simulink model "quad_sim_pyramid_formation"  (R2017b)
settings: Solver=VariableStepAuto  StartTime=0.0  StopTime=300  FixedStep=0.025  MaxStep=0.03  MinStep=0.02  RelTol=1e-3  EnableMultiTasking=on
InitFcn:
  | time_to_enable=250
  | 
  | setup_gains
  | % --- Outer loop gains --------
  | %P_X=9.44;   I_X=0.23;  D_X=2.36;
  | %P_Y=9.33;   I_Y=0.18;  D_Y=1.54;
  | % --------------------------
  | 
  | %CARLA TUNNED PID
  | %P_Z = 51.037;       I_Z = 43.051;        D_Z = 11.771;
  | %P_Z = 0.5;       I_Z = 0.15;        D_Z = 0.2;
  | %P_Z = 32.55;       I_Z = 9.82;        D_Z = 4.65 ;
  | 
  | global clientID;
  | clientID=-1;
values from neighbouring files (symbols this model uses):
  End_POS_pyramid = End_POS_pyramid*0.9995    [sim_formation_syscon.m]    (also in sim_formation_syscon_vel.m = End_POS_pyramid*0.999; structure_assembly.m = End_POS_pyramid*0.995)
undefined symbols (not defined in the file or in its folder): Kd_az, Kd_px, Kd_py, Kd_pz, Kd_vx, Kd_vy, Kd_vz, Ki_az, Ki_px, Ki_py, Ki_pz, Ki_vx, Ki_vy, Ki_vz, Kp_az, Kp_px, Kp_py, Kp_pz, Kp_vx, Kp_vy, Kp_vz, Start_POS, W, X, Y, Z
libraries: robotlib x27, dspsigops x27, simulink x27, dspindex x9
(part 3 of 3)

== system quad_sim_pyramid_formation/Quadrotor 5/Quadrirrotor Communication ==
  roll : Inport
  pitch : Inport  Port=2
  yaw : Inport  Port=3
  throttle : Inport  Port=4
  Blank Message : robotlib/Blank Message  SourceLibraryInfo=This block requires Robotics System Toolbox  messageType=geometry_msgs/Quaternion  SampleTime=inf
      settings: SourceProductBaseCode=RO
  Bus Assignment1 : BusAssignment  DialogController=Simulink.DDGSource_BusAssignment  AssignedSignals=X,Y,Z,W
  Bus Selector1 : BusSelector  OutputSignals=Data
  Data Type Conversion : DataTypeConversion  OutDataTypeStr=double
  Multiport Selector : dspindex/Multiport Selector  rowsOrCols=Rows  idxCellArray={ 1,2,3,4,5,6,7,8,9}  idxErrMode=Generate Error
  Publish2 : robotlib/Publish  SourceLibraryInfo=This block requires Robotics System Toolbox  topicSource=Specify your own  topic=/commands_attitude_5  messageType=geometry_msgs/Quaternion  messageQueueLength=105
      settings: SourceProductBaseCode=RO
  Subscribe : robotlib/Subscribe  SourceLibraryInfo=This block requires Robotics System Toolbox  topicSource=Specify your own  topic=/quadrotor_states_5  messageType=std_msgs/Float32MultiArray  sampleTime=-1  messageQueueLength=51
      settings: SourceProductBaseCode=RO
  Terminator : Terminator
  quad_pos_x : Outport
  quad_pos_y : Outport  Port=2
  quad_pos_z : Outport  Port=3
  quad_vel_x : Outport  Port=4
  quad_vel_y : Outport  Port=5
  quad_vel_z : Outport  Port=6
  quad_acc_x : Outport  Port=7
  quad_acc_y : Outport  Port=8
  quad_acc_z : Outport  Port=9
  wires:
  Blank Message/1 -> Bus Assignment1/1
  Subscribe/1 -> Terminator/1
  Subscribe/2 -> Bus Selector1/1
  Bus Assignment1/1 -> Publish2/1
  Multiport Selector/1 -> quad_pos_x/1
  Multiport Selector/2 -> quad_pos_y/1
  Multiport Selector/3 -> quad_pos_z/1
  Multiport Selector/4 -> quad_vel_x/1
  Multiport Selector/5 -> quad_vel_y/1
  Multiport Selector/6 -> quad_vel_z/1
  Multiport Selector/7 -> quad_acc_x/1
  Multiport Selector/8 -> quad_acc_y/1
  Multiport Selector/9 -> quad_acc_z/1
  Data Type Conversion/1 -> Multiport Selector/1
  Bus Selector1/1 -> Data Type Conversion/1  "<Data>"
  throttle/1 -> Bus Assignment1/5
  yaw/1 -> Bus Assignment1/4
  pitch/1 -> Bus Assignment1/3
  roll/1 -> Bus Assignment1/2

== system quad_sim_pyramid_formation/Quadrotor 5/Subsystem1 ==
  desired : Inport
  actual : Inport  Port=2
  roll_in : Inport  Port=3
  pitch_in : Inport  Port=4
  yaw_in : Inport  Port=5
  height_in : Inport  Port=6
  Clock : Clock
  Compare To Constant : simulink/Logic and Bit Operations/Compare To Constant  relop=<  const=0.5  OutDataTypeStr=boolean
  Compare To Constant1 : simulink/Logic and Bit Operations/Compare To Constant  relop=<=  const=0.025  OutDataTypeStr=boolean
  Compare To Zero : simulink/Logic and Bit Operations/Compare To Zero  relop=<=  OutDataTypeStr=boolean
  Constant : Constant  Value=0
  Constant1 : Constant
  Data Store Memory : DataStoreMemory  DataStoreName=waypoints_reached5  ShowAdditionalParam=off  OutDataTypeStr=boolean
  Data Store Read{,1..4} (5 alike) : DataStoreRead  DataStoreName=waypoints_reached5
  Data Store Write : DataStoreWrite  DataStoreName=waypoints_reached5
  Demux : Demux  Outputs=3
  Fcn : Fcn  Expr=sqrt(u(1)^2+u(2)^2+u(3)^2)
  Logical Operator : Logic  AllPortsSameDT=off  OutDataTypeStr=boolean
  Mux8 : Mux  Inputs=3
  Sum1 : Sum  Inputs=+-
  Switch{,1..4} (5 alike) : Switch  Criteria=u2 > Threshold  Threshold=0.5
  Switch5 : Switch  Criteria=u2 > Threshold  Threshold=time_to_enable
  "angle " : Constant  Value=0
  angle 1 : Constant  Value=0
  angle 2 : Constant  Value=0
  angle 3 : Constant  Value=-1
  roll_out : Outport
  pitch_out : Outport  Port=2
  yaw_out : Outport  Port=3
  height_out : Outport  Port=4
  wires:
  roll_in/1 -> Switch1/3
  pitch_in/1 -> Switch2/3
  angle 2/1 -> Switch3/1
  yaw_in/1 -> Switch3/3
  "angle "/1 -> Switch1/1
  angle 1/1 -> Switch2/1
  height_in/1 -> Switch4/3
  Switch2/1 -> pitch_out/1
  Switch1/1 -> roll_out/1
  Demux/2 -> Mux8/2
  Demux/3 -> Switch5/1, Mux8/3
  Logical Operator/1 -> Switch/3
  Compare To Constant/1 -> Logical Operator/1
  Compare To Constant1/1 -> Logical Operator/2
  Sum1/1 -> Fcn/1
  Fcn/1 -> Compare To Constant1/1
  Mux8/1 -> Sum1/1
  Compare To Zero/1 -> Switch/1
  Data Store Read2/1 -> Switch2/2
  Data Store Read4/1 -> Switch4/2
  Data Store Read1/1 -> Switch1/2
  Switch/1 -> Data Store Write/1
  Data Store Read3/1 -> Switch3/2
  angle 3/1 -> Switch4/1
  Switch3/1 -> yaw_out/1
  Switch4/1 -> height_out/1
  Data Store Read/1 -> Switch/2
  Constant/1 -> Compare To Zero/1
  Demux/1 -> Mux8/1
  desired/1 -> Demux/1
  actual/1 -> Sum1/2
  Clock/1 -> Switch5/2
  Constant1/1 -> Switch5/3
  Switch5/1 -> Compare To Constant/1

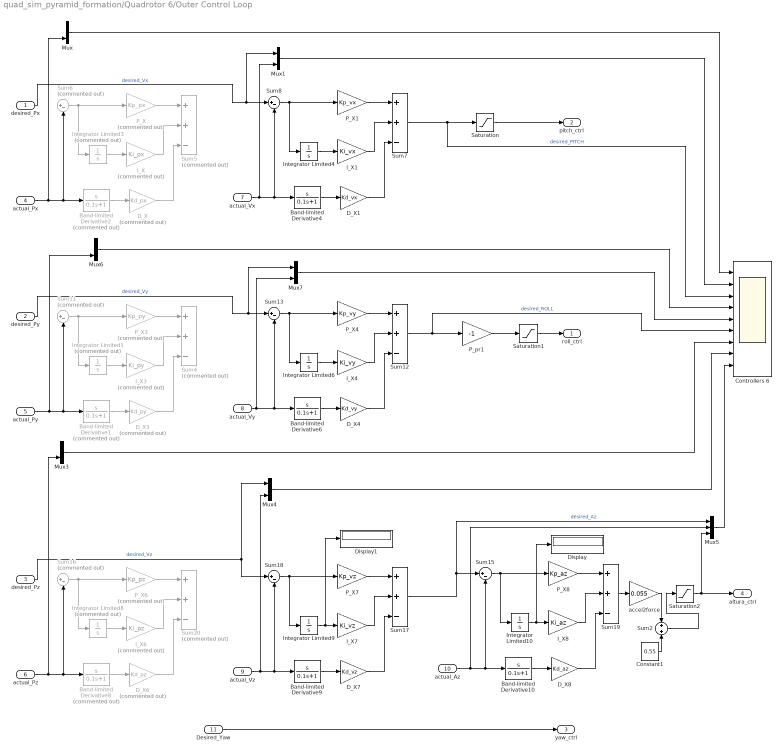
== system quad_sim_pyramid_formation/Quadrotor 6/Outer Control Loop ==
  desired_Px : Inport
  desired_Py : Inport  Port=2
  desired_Pz : Inport  Port=3
  actual_Px : Inport  Port=4
  actual_Py : Inport  Port=5
  actual_Pz : Inport  Port=6
  actual_Vx : Inport  Port=7
  actual_Vy : Inport  Port=8
  actual_Vz : Inport  Port=9
  actual_Az : Inport  Port=10
  Desired_Yaw : Inport  Port=11
  Band-limited Derivative1 : TransferFcn  Commented=on  Numerator=[1 0]  Denominator=[0.1 1]
  Band-limited Derivative{4,6,9..10} (4 alike) : TransferFcn  Numerator=[1 0]  Denominator=[0.1 1]
  Band-limited Derivative2 : TransferFcn  Commented=on  Numerator=[1 0]  Denominator=[0.1 1]
  Band-limited Derivative8 : TransferFcn  Commented=on  Numerator=[1 0]  Denominator=[0.1 1]
  Constant1 : Constant  Value=0.55
  Controllers 6 : Scope  NumInputPorts=9
  D_X : Gain  Commented=on  Gain=Kd_px
  D_X1 : Gain  Gain=Kd_vx
  D_X3 : Gain  Commented=on  Gain=Kd_py
  D_X4 : Gain  Gain=Kd_vy
  D_X6 : Gain  Commented=on  Gain=Kd_pz
  D_X7 : Gain  Gain=Kd_vz
  D_X8 : Gain  Gain=Kd_az
  Display : Display
  Display1 : Display
  I_X : Gain  Commented=on  Gain=Ki_px
  I_X1 : Gain  Gain=Ki_vx
  I_X3 : Gain  Commented=on  Gain=Ki_py
  I_X4 : Gain  Gain=Ki_vy
  I_X6 : Gain  Commented=on  Gain=Ki_pz
  I_X7 : Gain  Gain=Ki_vz
  I_X8 : Gain  Gain=Ki_az
  Integrator Limited1 : Integrator  Commented=on  LimitOutput=on  UpperSaturationLimit=100  LowerSaturationLimit=-100
  Integrator Limited10 : Integrator  LimitOutput=on  UpperSaturationLimit=1000  LowerSaturationLimit=-1000
  Integrator Limited3 : Integrator  Commented=on  LimitOutput=on  UpperSaturationLimit=100  LowerSaturationLimit=-100
  Integrator Limited4 : Integrator  LimitOutput=on  UpperSaturationLimit=100  LowerSaturationLimit=-100
  Integrator Limited6 : Integrator  LimitOutput=on  UpperSaturationLimit=100  LowerSaturationLimit=-100
  Integrator Limited8 : Integrator  Commented=on  LimitOutput=on  UpperSaturationLimit=1000  LowerSaturationLimit=-1000
  Integrator Limited9 : Integrator  LimitOutput=on  UpperSaturationLimit=1000  LowerSaturationLimit=-1000
  Mux{,1,3..4,6..7} (6 alike) : Mux  Inputs=2
  Mux5 : Mux  Inputs=3
  P_X : Gain  Commented=on  Gain=Kp_px
  P_X1 : Gain  Gain=Kp_vx
  P_X3 : Gain  Commented=on  Gain=Kp_py
  P_X4 : Gain  Gain=Kp_vy
  P_X6 : Gain  Commented=on  Gain=Kp_pz
  P_X7 : Gain  Gain=Kp_vz
  P_X8 : Gain  Gain=Kp_az
  P_pr1 : Gain  Gain=-1
  Saturation : Saturate  UpperLimit=5  LowerLimit=-5
  Saturation1 : Saturate  UpperLimit=5  LowerLimit=-5
  Saturation2 : Saturate  UpperLimit=10  LowerLimit=0
  Sum11 : Sum  Commented=on  Inputs=|+-
  Sum{7,12,17,19} (4 alike) : Sum  Inputs=++-
  Sum{8,13,15,18} (4 alike) : Sum  Inputs=|+-
  Sum16 : Sum  Commented=on  Inputs=|+-
  Sum2 : Sum  Inputs=+|+
  Sum20 : Sum  Commented=on  Inputs=++-
  Sum4 : Sum  Commented=on  Inputs=++-
  Sum5 : Sum  Commented=on  Inputs=++-
  Sum6 : Sum  Commented=on  Inputs=|+-
  accel2force : Gain  Gain=0.055
  roll_ctrl : Outport
  pitch_ctrl : Outport  Port=2
  yaw_ctrl : Outport  Port=3
  altura_ctrl : Outport  Port=4
  wires:
  Saturation1/1 -> roll_ctrl/1
  Saturation/1 -> pitch_ctrl/1
  P_pr1/1 -> Saturation1/1
  Mux7/1 -> Controllers 6/5
  Mux6/1 -> Controllers 6/4
  actual_Vy/1 -> Mux7/2, Sum13/2, Band-limited Derivative6/1
  actual_Py/1 -> Mux6/2, Band-limited Derivative1/1, Sum11/2
  Constant1/1 -> Sum2/2
  accel2force/1 -> Sum2/1
  Sum2/1 -> Saturation2/1
  Sum19/1 -> accel2force/1
  Mux5/1 -> Controllers 6/9
  Mux4/1 -> Controllers 6/8
  Mux3/1 -> Controllers 6/7
  Sum17/1 -> Sum15/1, Mux5/1  "desired_Az"
  actual_Az/1 -> Sum15/2, Band-limited Derivative10/1, Mux5/2
  desired_Pz/1 -> Sum18/1, Mux4/1  "desired_Vz"
  actual_Vz/1 -> Band-limited Derivative9/1, Sum18/2, Mux4/2
  Mux1/1 -> Controllers 6/2
  Mux/1 -> Controllers 6/1
  I_X8/1 -> Sum19/2
  Band-limited Derivative10/1 -> D_X8/1
  D_X8/1 -> Sum19/3
  P_X8/1 -> Sum19/1
  Integrator Limited10/1 -> I_X8/1, Display/1
  Sum15/1 -> P_X8/1, Integrator Limited10/1
  I_X7/1 -> Sum17/2
  Band-limited Derivative9/1 -> D_X7/1
  D_X7/1 -> Sum17/3
  P_X7/1 -> Sum17/1
  Integrator Limited9/1 -> I_X7/1, Display1/1
  Sum18/1 -> Integrator Limited9/1, P_X7/1
  I_X6/1 -> Sum20/2
  Band-limited Derivative8/1 -> D_X6/1
  actual_Pz/1 -> Sum16/2, Band-limited Derivative8/1, Mux3/2
  D_X6/1 -> Sum20/3
  P_X6/1 -> Sum20/1
  Integrator Limited8/1 -> I_X6/1
  Sum16/1 -> P_X6/1, Integrator Limited8/1
  Sum12/1 -> Controllers 6/6, P_pr1/1  "desired_ROLL"
  desired_Py/1 -> Mux7/1, Sum13/1  "desired_Vy"
  I_X4/1 -> Sum12/2
  Band-limited Derivative6/1 -> D_X4/1
  D_X4/1 -> Sum12/3
  P_X4/1 -> Sum12/1
  Integrator Limited6/1 -> I_X4/1
  Sum13/1 -> P_X4/1, Integrator Limited6/1
  I_X3/1 -> Sum4/2
  Band-limited Derivative1/1 -> D_X3/1
  D_X3/1 -> Sum4/3
  P_X3/1 -> Sum4/1
  Integrator Limited1/1 -> I_X3/1
  Sum11/1 -> Integrator Limited1/1, P_X3/1
  Sum7/1 -> Controllers 6/3, Saturation/1  "desired_PITCH"
  desired_Px/1 -> Sum8/1, Mux1/1  "desired_Vx"
  I_X1/1 -> Sum7/2
  Band-limited Derivative4/1 -> D_X1/1
  actual_Vx/1 -> Band-limited Derivative4/1, Sum8/2, Mux1/2
  D_X1/1 -> Sum7/3
  P_X1/1 -> Sum7/1
  Integrator Limited4/1 -> I_X1/1
  Sum8/1 -> Integrator Limited4/1, P_X1/1
  Saturation2/1 -> altura_ctrl/1, Mux5/3
  I_X/1 -> Sum5/2
  Band-limited Derivative2/1 -> D_X/1
  actual_Px/1 -> Sum6/2, Band-limited Derivative2/1, Mux/2
  D_X/1 -> Sum5/3
  P_X/1 -> Sum5/1
  Integrator Limited3/1 -> I_X/1
  Sum6/1 -> P_X/1, Integrator Limited3/1
  Desired_Yaw/1 -> yaw_ctrl/1

== system quad_sim_pyramid_formation/Quadrotor 6/Quadrirrotor Communication ==
  roll : Inport
  pitch : Inport  Port=2
  yaw : Inport  Port=3
  throttle : Inport  Port=4
  Blank Message : robotlib/Blank Message  SourceLibraryInfo=This block requires Robotics System Toolbox  messageType=geometry_msgs/Quaternion  SampleTime=inf
      settings: SourceProductBaseCode=RO
  Bus Assignment1 : BusAssignment  DialogController=Simulink.DDGSource_BusAssignment  AssignedSignals=X,Y,Z,W
  Bus Selector1 : BusSelector  OutputSignals=Data
  Data Type Conversion : DataTypeConversion  OutDataTypeStr=double
  Multiport Selector : dspindex/Multiport Selector  rowsOrCols=Rows  idxCellArray={ 1,2,3,4,5,6,7,8,9}  idxErrMode=Generate Error
  Publish2 : robotlib/Publish  SourceLibraryInfo=This block requires Robotics System Toolbox  topicSource=Specify your own  topic=/commands_attitude_6  messageType=geometry_msgs/Quaternion  messageQueueLength=105
      settings: SourceProductBaseCode=RO
  Subscribe : robotlib/Subscribe  SourceLibraryInfo=This block requires Robotics System Toolbox  topicSource=Specify your own  topic=/quadrotor_states_6  messageType=std_msgs/Float32MultiArray  sampleTime=-1  messageQueueLength=51
      settings: SourceProductBaseCode=RO
  Terminator : Terminator
  quad_pos_x : Outport
  quad_pos_y : Outport  Port=2
  quad_pos_z : Outport  Port=3
  quad_vel_x : Outport  Port=4
  quad_vel_y : Outport  Port=5
  quad_vel_z : Outport  Port=6
  quad_acc_x : Outport  Port=7
  quad_acc_y : Outport  Port=8
  quad_acc_z : Outport  Port=9
  wires:
  roll/1 -> Bus Assignment1/2
  pitch/1 -> Bus Assignment1/3
  yaw/1 -> Bus Assignment1/4
  throttle/1 -> Bus Assignment1/5
  Bus Selector1/1 -> Data Type Conversion/1  "<Data>"
  Data Type Conversion/1 -> Multiport Selector/1
  Multiport Selector/9 -> quad_acc_z/1
  Multiport Selector/8 -> quad_acc_y/1
  Multiport Selector/7 -> quad_acc_x/1
  Multiport Selector/6 -> quad_vel_z/1
  Multiport Selector/5 -> quad_vel_y/1
  Multiport Selector/4 -> quad_vel_x/1
  Multiport Selector/3 -> quad_pos_z/1
  Multiport Selector/2 -> quad_pos_y/1
  Multiport Selector/1 -> quad_pos_x/1
  Bus Assignment1/1 -> Publish2/1
  Subscribe/2 -> Bus Selector1/1
  Subscribe/1 -> Terminator/1
  Blank Message/1 -> Bus Assignment1/1

== system quad_sim_pyramid_formation/Quadrotor 6/Subsystem1 ==
  desired : Inport
  actual : Inport  Port=2
  roll_in : Inport  Port=3
  pitch_in : Inport  Port=4
  yaw_in : Inport  Port=5
  height_in : Inport  Port=6
  Clock : Clock
  Compare To Constant : simulink/Logic and Bit Operations/Compare To Constant  relop=<  const=0.5  OutDataTypeStr=boolean
  Compare To Constant1 : simulink/Logic and Bit Operations/Compare To Constant  relop=<=  const=0.025  OutDataTypeStr=boolean
  Compare To Zero : simulink/Logic and Bit Operations/Compare To Zero  relop=<=  OutDataTypeStr=boolean
  Constant : Constant  Value=0
  Constant1 : Constant
  Data Store Memory : DataStoreMemory  DataStoreName=waypoints_reached6  ShowAdditionalParam=off  OutDataTypeStr=boolean
  Data Store Read{,1..4} (5 alike) : DataStoreRead  DataStoreName=waypoints_reached6
  Data Store Write : DataStoreWrite  DataStoreName=waypoints_reached6
  Demux : Demux  Outputs=3
  Fcn : Fcn  Expr=sqrt(u(1)^2+u(2)^2+u(3)^2)
  Logical Operator : Logic  AllPortsSameDT=off  OutDataTypeStr=boolean
  Mux8 : Mux  Inputs=3
  Sum1 : Sum  Inputs=+-
  Switch{,1..4} (5 alike) : Switch  Criteria=u2 > Threshold  Threshold=0.5
  Switch5 : Switch  Criteria=u2 > Threshold  Threshold=time_to_enable
  "angle " : Constant  Value=0
  angle 1 : Constant  Value=0
  angle 2 : Constant  Value=0
  angle 3 : Constant  Value=-1
  roll_out : Outport
  pitch_out : Outport  Port=2
  yaw_out : Outport  Port=3
  height_out : Outport  Port=4
  wires:
  roll_in/1 -> Switch1/3
  pitch_in/1 -> Switch2/3
  angle 2/1 -> Switch3/1
  yaw_in/1 -> Switch3/3
  "angle "/1 -> Switch1/1
  angle 1/1 -> Switch2/1
  height_in/1 -> Switch4/3
  Switch2/1 -> pitch_out/1
  Switch1/1 -> roll_out/1
  Demux/2 -> Mux8/2
  Demux/3 -> Switch5/1, Mux8/3
  Logical Operator/1 -> Switch/3
  Compare To Constant/1 -> Logical Operator/1
  Compare To Constant1/1 -> Logical Operator/2
  Sum1/1 -> Fcn/1
  Fcn/1 -> Compare To Constant1/1
  Mux8/1 -> Sum1/1
  Compare To Zero/1 -> Switch/1
  Data Store Read2/1 -> Switch2/2
  Data Store Read4/1 -> Switch4/2
  Data Store Read1/1 -> Switch1/2
  Switch/1 -> Data Store Write/1
  Data Store Read3/1 -> Switch3/2
  angle 3/1 -> Switch4/1
  Switch3/1 -> yaw_out/1
  Switch4/1 -> height_out/1
  Data Store Read/1 -> Switch/2
  Constant/1 -> Compare To Zero/1
  Demux/1 -> Mux8/1
  desired/1 -> Demux/1
  actual/1 -> Sum1/2
  Clock/1 -> Switch5/2
  Constant1/1 -> Switch5/3
  Switch5/1 -> Compare To Constant/1

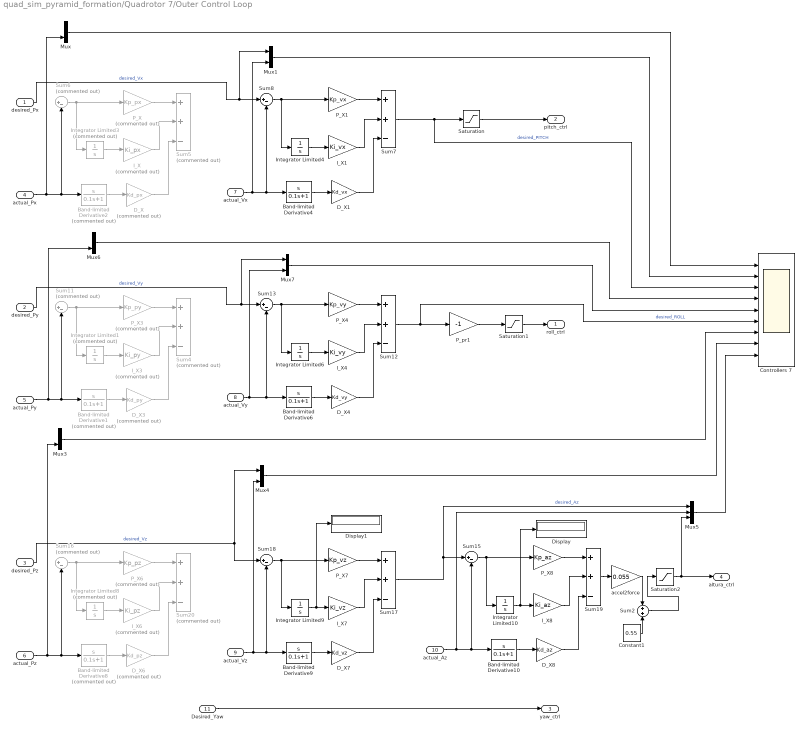
== system quad_sim_pyramid_formation/Quadrotor 7/Outer Control Loop ==
  desired_Px : Inport
  desired_Py : Inport  Port=2
  desired_Pz : Inport  Port=3
  actual_Px : Inport  Port=4
  actual_Py : Inport  Port=5
  actual_Pz : Inport  Port=6
  actual_Vx : Inport  Port=7
  actual_Vy : Inport  Port=8
  actual_Vz : Inport  Port=9
  actual_Az : Inport  Port=10
  Desired_Yaw : Inport  Port=11
  Band-limited Derivative1 : TransferFcn  Commented=on  Numerator=[1 0]  Denominator=[0.1 1]
  Band-limited Derivative{4,6,9..10} (4 alike) : TransferFcn  Numerator=[1 0]  Denominator=[0.1 1]
  Band-limited Derivative2 : TransferFcn  Commented=on  Numerator=[1 0]  Denominator=[0.1 1]
  Band-limited Derivative8 : TransferFcn  Commented=on  Numerator=[1 0]  Denominator=[0.1 1]
  Constant1 : Constant  Value=0.55
  Controllers 7 : Scope  NumInputPorts=9
  D_X : Gain  Commented=on  Gain=Kd_px
  D_X1 : Gain  Gain=Kd_vx
  D_X3 : Gain  Commented=on  Gain=Kd_py
  D_X4 : Gain  Gain=Kd_vy
  D_X6 : Gain  Commented=on  Gain=Kd_pz
  D_X7 : Gain  Gain=Kd_vz
  D_X8 : Gain  Gain=Kd_az
  Display : Display
  Display1 : Display
  I_X : Gain  Commented=on  Gain=Ki_px
  I_X1 : Gain  Gain=Ki_vx
  I_X3 : Gain  Commented=on  Gain=Ki_py
  I_X4 : Gain  Gain=Ki_vy
  I_X6 : Gain  Commented=on  Gain=Ki_pz
  I_X7 : Gain  Gain=Ki_vz
  I_X8 : Gain  Gain=Ki_az
  Integrator Limited1 : Integrator  Commented=on  LimitOutput=on  UpperSaturationLimit=100  LowerSaturationLimit=-100
  Integrator Limited10 : Integrator  LimitOutput=on  UpperSaturationLimit=1000  LowerSaturationLimit=-1000
  Integrator Limited3 : Integrator  Commented=on  LimitOutput=on  UpperSaturationLimit=100  LowerSaturationLimit=-100
  Integrator Limited4 : Integrator  LimitOutput=on  UpperSaturationLimit=100  LowerSaturationLimit=-100
  Integrator Limited6 : Integrator  LimitOutput=on  UpperSaturationLimit=100  LowerSaturationLimit=-100
  Integrator Limited8 : Integrator  Commented=on  LimitOutput=on  UpperSaturationLimit=1000  LowerSaturationLimit=-1000
  Integrator Limited9 : Integrator  LimitOutput=on  UpperSaturationLimit=1000  LowerSaturationLimit=-1000
  Mux{,1,3..4,6..7} (6 alike) : Mux  Inputs=2
  Mux5 : Mux  Inputs=3
  P_X : Gain  Commented=on  Gain=Kp_px
  P_X1 : Gain  Gain=Kp_vx
  P_X3 : Gain  Commented=on  Gain=Kp_py
  P_X4 : Gain  Gain=Kp_vy
  P_X6 : Gain  Commented=on  Gain=Kp_pz
  P_X7 : Gain  Gain=Kp_vz
  P_X8 : Gain  Gain=Kp_az
  P_pr1 : Gain  Gain=-1
  Saturation : Saturate  UpperLimit=5  LowerLimit=-5
  Saturation1 : Saturate  UpperLimit=5  LowerLimit=-5
  Saturation2 : Saturate  UpperLimit=10  LowerLimit=0
  Sum11 : Sum  Commented=on  Inputs=|+-
  Sum{7,12,17,19} (4 alike) : Sum  Inputs=++-
  Sum{8,13,15,18} (4 alike) : Sum  Inputs=|+-
  Sum16 : Sum  Commented=on  Inputs=|+-
  Sum2 : Sum  Inputs=+|+
  Sum20 : Sum  Commented=on  Inputs=++-
  Sum4 : Sum  Commented=on  Inputs=++-
  Sum5 : Sum  Commented=on  Inputs=++-
  Sum6 : Sum  Commented=on  Inputs=|+-
  accel2force : Gain  Gain=0.055
  roll_ctrl : Outport
  pitch_ctrl : Outport  Port=2
  yaw_ctrl : Outport  Port=3
  altura_ctrl : Outport  Port=4
  wires:
  Desired_Yaw/1 -> yaw_ctrl/1
  Sum6/1 -> Integrator Limited3/1, P_X/1
  Integrator Limited3/1 -> I_X/1
  P_X/1 -> Sum5/1
  D_X/1 -> Sum5/3
  actual_Px/1 -> Mux/2, Band-limited Derivative2/1, Sum6/2
  Band-limited Derivative2/1 -> D_X/1
  I_X/1 -> Sum5/2
  Saturation2/1 -> Mux5/3, altura_ctrl/1
  Sum8/1 -> P_X1/1, Integrator Limited4/1
  Integrator Limited4/1 -> I_X1/1
  P_X1/1 -> Sum7/1
  D_X1/1 -> Sum7/3
  actual_Vx/1 -> Mux1/2, Sum8/2, Band-limited Derivative4/1
  Band-limited Derivative4/1 -> D_X1/1
  I_X1/1 -> Sum7/2
  desired_Px/1 -> Mux1/1, Sum8/1  "desired_Vx"
  Sum7/1 -> Controllers 7/3, Saturation/1  "desired_PITCH"
  Sum11/1 -> P_X3/1, Integrator Limited1/1
  Integrator Limited1/1 -> I_X3/1
  P_X3/1 -> Sum4/1
  D_X3/1 -> Sum4/3
  Band-limited Derivative1/1 -> D_X3/1
  I_X3/1 -> Sum4/2
  Sum13/1 -> Integrator Limited6/1, P_X4/1
  Integrator Limited6/1 -> I_X4/1
  P_X4/1 -> Sum12/1
  D_X4/1 -> Sum12/3
  Band-limited Derivative6/1 -> D_X4/1
  I_X4/1 -> Sum12/2
  desired_Py/1 -> Sum13/1, Mux7/1  "desired_Vy"
  Sum12/1 -> Controllers 7/6, P_pr1/1  "desired_ROLL"
  Sum16/1 -> Integrator Limited8/1, P_X6/1
  Integrator Limited8/1 -> I_X6/1
  P_X6/1 -> Sum20/1
  D_X6/1 -> Sum20/3
  actual_Pz/1 -> Mux3/2, Band-limited Derivative8/1, Sum16/2
  Band-limited Derivative8/1 -> D_X6/1
  I_X6/1 -> Sum20/2
  Sum18/1 -> P_X7/1, Integrator Limited9/1
  Integrator Limited9/1 -> Display1/1, I_X7/1
  P_X7/1 -> Sum17/1
  D_X7/1 -> Sum17/3
  Band-limited Derivative9/1 -> D_X7/1
  I_X7/1 -> Sum17/2
  Sum15/1 -> Integrator Limited10/1, P_X8/1
  Integrator Limited10/1 -> Display/1, I_X8/1
  P_X8/1 -> Sum19/1
  D_X8/1 -> Sum19/3
  Band-limited Derivative10/1 -> D_X8/1
  I_X8/1 -> Sum19/2
  Mux/1 -> Controllers 7/1
  Mux1/1 -> Controllers 7/2
  actual_Vz/1 -> Mux4/2, Sum18/2, Band-limited Derivative9/1
  desired_Pz/1 -> Sum18/1, Mux4/1  "desired_Vz"
  actual_Az/1 -> Mux5/2, Band-limited Derivative10/1, Sum15/2
  Sum17/1 -> Mux5/1, Sum15/1  "desired_Az"
  Mux3/1 -> Controllers 7/7
  Mux4/1 -> Controllers 7/8
  Mux5/1 -> Controllers 7/9
  Sum19/1 -> accel2force/1
  Sum2/1 -> Saturation2/1
  accel2force/1 -> Sum2/1
  Constant1/1 -> Sum2/2
  actual_Py/1 -> Sum11/2, Band-limited Derivative1/1, Mux6/2
  actual_Vy/1 -> Band-limited Derivative6/1, Sum13/2, Mux7/2
  Mux6/1 -> Controllers 7/4
  Mux7/1 -> Controllers 7/5
  P_pr1/1 -> Saturation1/1
  Saturation/1 -> pitch_ctrl/1
  Saturation1/1 -> roll_ctrl/1

== system quad_sim_pyramid_formation/Quadrotor 7/Quadrirrotor Communication ==
  roll : Inport
  pitch : Inport  Port=2
  yaw : Inport  Port=3
  throttle : Inport  Port=4
  Blank Message : robotlib/Blank Message  SourceLibraryInfo=This block requires Robotics System Toolbox  messageType=geometry_msgs/Quaternion  SampleTime=inf
      settings: SourceProductBaseCode=RO
  Bus Assignment1 : BusAssignment  DialogController=Simulink.DDGSource_BusAssignment  AssignedSignals=X,Y,Z,W
  Bus Selector1 : BusSelector  OutputSignals=Data
  Data Type Conversion : DataTypeConversion  OutDataTypeStr=double
  Multiport Selector : dspindex/Multiport Selector  rowsOrCols=Rows  idxCellArray={ 1,2,3,4,5,6,7,8,9}  idxErrMode=Generate Error
  Publish2 : robotlib/Publish  SourceLibraryInfo=This block requires Robotics System Toolbox  topicSource=Specify your own  topic=/commands_attitude_7  messageType=geometry_msgs/Quaternion  messageQueueLength=105
      settings: SourceProductBaseCode=RO
  Subscribe : robotlib/Subscribe  SourceLibraryInfo=This block requires Robotics System Toolbox  topicSource=Specify your own  topic=/quadrotor_states_7  messageType=std_msgs/Float32MultiArray  sampleTime=-1  messageQueueLength=51
      settings: SourceProductBaseCode=RO
  Terminator : Terminator
  quad_pos_x : Outport
  quad_pos_y : Outport  Port=2
  quad_pos_z : Outport  Port=3
  quad_vel_x : Outport  Port=4
  quad_vel_y : Outport  Port=5
  quad_vel_z : Outport  Port=6
  quad_acc_x : Outport  Port=7
  quad_acc_y : Outport  Port=8
  quad_acc_z : Outport  Port=9
  wires:
  Blank Message/1 -> Bus Assignment1/1
  Subscribe/1 -> Terminator/1
  Subscribe/2 -> Bus Selector1/1
  Bus Assignment1/1 -> Publish2/1
  Multiport Selector/1 -> quad_pos_x/1
  Multiport Selector/2 -> quad_pos_y/1
  Multiport Selector/3 -> quad_pos_z/1
  Multiport Selector/4 -> quad_vel_x/1
  Multiport Selector/5 -> quad_vel_y/1
  Multiport Selector/6 -> quad_vel_z/1
  Multiport Selector/7 -> quad_acc_x/1
  Multiport Selector/8 -> quad_acc_y/1
  Multiport Selector/9 -> quad_acc_z/1
  Data Type Conversion/1 -> Multiport Selector/1
  Bus Selector1/1 -> Data Type Conversion/1  "<Data>"
  throttle/1 -> Bus Assignment1/5
  yaw/1 -> Bus Assignment1/4
  pitch/1 -> Bus Assignment1/3
  roll/1 -> Bus Assignment1/2

== system quad_sim_pyramid_formation/Quadrotor 7/Subsystem1 ==
  desired : Inport
  actual : Inport  Port=2
  roll_in : Inport  Port=3
  pitch_in : Inport  Port=4
  yaw_in : Inport  Port=5
  height_in : Inport  Port=6
  Clock : Clock
  Compare To Constant : simulink/Logic and Bit Operations/Compare To Constant  relop=<  const=0.5  OutDataTypeStr=boolean
  Compare To Constant1 : simulink/Logic and Bit Operations/Compare To Constant  relop=<=  const=0.025  OutDataTypeStr=boolean
  Compare To Zero : simulink/Logic and Bit Operations/Compare To Zero  relop=<=  OutDataTypeStr=boolean
  Constant : Constant  Value=0
  Constant1 : Constant
  Data Store Memory : DataStoreMemory  DataStoreName=waypoints_reached7  ShowAdditionalParam=off  OutDataTypeStr=boolean
  Data Store Read{,1..4} (5 alike) : DataStoreRead  DataStoreName=waypoints_reached7
  Data Store Write : DataStoreWrite  DataStoreName=waypoints_reached7
  Demux : Demux  Outputs=3
  Fcn : Fcn  Expr=sqrt(u(1)^2+u(2)^2+u(3)^2)
  Logical Operator : Logic  AllPortsSameDT=off  OutDataTypeStr=boolean
  Mux8 : Mux  Inputs=3
  Sum1 : Sum  Inputs=+-
  Switch{,1..4} (5 alike) : Switch  Criteria=u2 > Threshold  Threshold=0.5
  Switch5 : Switch  Criteria=u2 > Threshold  Threshold=time_to_enable
  "angle " : Constant  Value=0
  angle 1 : Constant  Value=0
  angle 2 : Constant  Value=0
  angle 3 : Constant  Value=-1
  roll_out : Outport
  pitch_out : Outport  Port=2
  yaw_out : Outport  Port=3
  height_out : Outport  Port=4
  wires:
  roll_in/1 -> Switch1/3
  pitch_in/1 -> Switch2/3
  angle 2/1 -> Switch3/1
  yaw_in/1 -> Switch3/3
  "angle "/1 -> Switch1/1
  angle 1/1 -> Switch2/1
  height_in/1 -> Switch4/3
  Switch2/1 -> pitch_out/1
  Switch1/1 -> roll_out/1
  Demux/2 -> Mux8/2
  Demux/3 -> Switch5/1, Mux8/3
  Logical Operator/1 -> Switch/3
  Compare To Constant/1 -> Logical Operator/1
  Compare To Constant1/1 -> Logical Operator/2
  Sum1/1 -> Fcn/1
  Fcn/1 -> Compare To Constant1/1
  Mux8/1 -> Sum1/1
  Compare To Zero/1 -> Switch/1
  Data Store Read2/1 -> Switch2/2
  Data Store Read4/1 -> Switch4/2
  Data Store Read1/1 -> Switch1/2
  Switch/1 -> Data Store Write/1
  Data Store Read3/1 -> Switch3/2
  angle 3/1 -> Switch4/1
  Switch3/1 -> yaw_out/1
  Switch4/1 -> height_out/1
  Data Store Read/1 -> Switch/2
  Constant/1 -> Compare To Zero/1
  Demux/1 -> Mux8/1
  desired/1 -> Demux/1
  actual/1 -> Sum1/2
  Clock/1 -> Switch5/2
  Constant1/1 -> Switch5/3
  Switch5/1 -> Compare To Constant/1

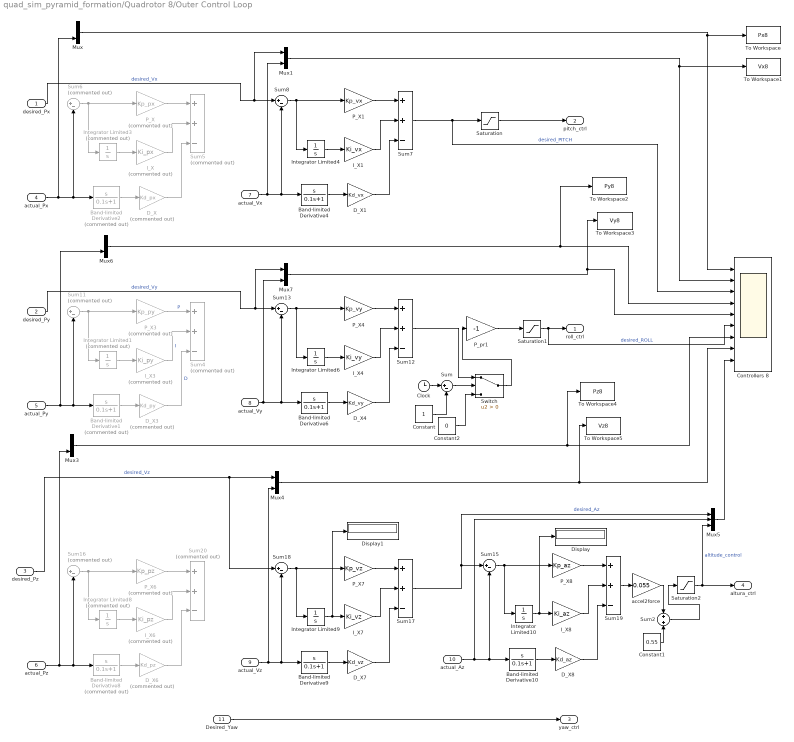
== system quad_sim_pyramid_formation/Quadrotor 8/Outer Control Loop ==
  desired_Px : Inport
  desired_Py : Inport  Port=2
  desired_Pz : Inport  Port=3
  actual_Px : Inport  Port=4
  actual_Py : Inport  Port=5
  actual_Pz : Inport  Port=6
  actual_Vx : Inport  Port=7
  actual_Vy : Inport  Port=8
  actual_Vz : Inport  Port=9
  actual_Az : Inport  Port=10
  Desired_Yaw : Inport  Port=11
  Band-limited Derivative1 : TransferFcn  Commented=on  Numerator=[1 0]  Denominator=[0.1 1]
  Band-limited Derivative{4,6,9..10} (4 alike) : TransferFcn  Numerator=[1 0]  Denominator=[0.1 1]
  Band-limited Derivative2 : TransferFcn  Commented=on  Numerator=[1 0]  Denominator=[0.1 1]
  Band-limited Derivative8 : TransferFcn  Commented=on  Numerator=[1 0]  Denominator=[0.1 1]
  Clock : Clock
  Constant : Constant
  Constant1 : Constant  Value=0.55
  Constant2 : Constant  Value=0
  Controllers 8 : Scope  NumInputPorts=9
  D_X : Gain  Commented=on  Gain=Kd_px
  D_X1 : Gain  Gain=Kd_vx
  D_X3 : Gain  Commented=on  Gain=Kd_py
  D_X4 : Gain  Gain=Kd_vy
  D_X6 : Gain  Commented=on  Gain=Kd_pz
  D_X7 : Gain  Gain=Kd_vz
  D_X8 : Gain  Gain=Kd_az
  Display : Display
  Display1 : Display
  I_X : Gain  Commented=on  Gain=Ki_px
  I_X1 : Gain  Gain=Ki_vx
  I_X3 : Gain  Commented=on  Gain=Ki_py
  I_X4 : Gain  Gain=Ki_vy
  I_X6 : Gain  Commented=on  Gain=Ki_pz
  I_X7 : Gain  Gain=Ki_vz
  I_X8 : Gain  Gain=Ki_az
  Integrator Limited1 : Integrator  Commented=on  LimitOutput=on  UpperSaturationLimit=100  LowerSaturationLimit=-100
  Integrator Limited10 : Integrator  LimitOutput=on  UpperSaturationLimit=1000  LowerSaturationLimit=-1000
  Integrator Limited3 : Integrator  Commented=on  LimitOutput=on  UpperSaturationLimit=100  LowerSaturationLimit=-100
  Integrator Limited4 : Integrator  LimitOutput=on  UpperSaturationLimit=100  LowerSaturationLimit=-100
  Integrator Limited6 : Integrator  LimitOutput=on  UpperSaturationLimit=100  LowerSaturationLimit=-100
  Integrator Limited8 : Integrator  Commented=on  LimitOutput=on  UpperSaturationLimit=1000  LowerSaturationLimit=-1000
  Integrator Limited9 : Integrator  LimitOutput=on  UpperSaturationLimit=1000  LowerSaturationLimit=-1000
  Mux{,1,3..4,6..7} (6 alike) : Mux  Inputs=2
  Mux5 : Mux  Inputs=3
  P_X : Gain  Commented=on  Gain=Kp_px
  P_X1 : Gain  Gain=Kp_vx
  P_X3 : Gain  Commented=on  Gain=Kp_py
  P_X4 : Gain  Gain=Kp_vy
  P_X6 : Gain  Commented=on  Gain=Kp_pz
  P_X7 : Gain  Gain=Kp_vz
  P_X8 : Gain  Gain=Kp_az
  P_pr1 : Gain  Gain=-1
  Saturation : Saturate  UpperLimit=5  LowerLimit=-5
  Saturation1 : Saturate  UpperLimit=5  LowerLimit=-5
  Saturation2 : Saturate  UpperLimit=10  LowerLimit=0
  Sum{,8,13,15,18} (5 alike) : Sum  Inputs=|+-
  Sum11 : Sum  Commented=on  Inputs=|+-
  Sum{7,12,17,19} (4 alike) : Sum  Inputs=++-
  Sum16 : Sum  Commented=on  Inputs=|+-
  Sum2 : Sum  Inputs=+|+
  Sum20 : Sum  Commented=on  Inputs=++-
  Sum4 : Sum  Commented=on  Inputs=++-
  Sum5 : Sum  Commented=on  Inputs=++-
  Sum6 : Sum  Commented=on  Inputs=|+-
  Switch : Switch  Criteria=u2 > Threshold
  To Workspace : ToWorkspace  VariableName=Px8  SaveFormat=Timeseries  SampleTime=-1
  To Workspace1 : ToWorkspace  VariableName=Vx8  SaveFormat=Timeseries  SampleTime=-1
  To Workspace2 : ToWorkspace  VariableName=Py8  SaveFormat=Timeseries  SampleTime=-1
  To Workspace3 : ToWorkspace  VariableName=Vy8  SaveFormat=Timeseries  SampleTime=-1
  To Workspace4 : ToWorkspace  VariableName=Pz8  SaveFormat=Timeseries  SampleTime=-1
  To Workspace5 : ToWorkspace  VariableName=Vz8  SaveFormat=Timeseries  SampleTime=-1
  accel2force : Gain  Gain=0.055
  roll_ctrl : Outport
  pitch_ctrl : Outport  Port=2
  yaw_ctrl : Outport  Port=3
  altura_ctrl : Outport  Port=4
  wires:
  Saturation1/1 -> Controllers 8/6, roll_ctrl/1  "desired_ROLL"
  Saturation/1 -> pitch_ctrl/1
  P_pr1/1 -> Saturation1/1
  Mux7/1 -> To Workspace3/1, Controllers 8/5
  Mux6/1 -> To Workspace2/1, Controllers 8/4
  actual_Vy/1 -> Mux7/2, Sum13/2, Band-limited Derivative6/1
  actual_Py/1 -> Mux6/2, Band-limited Derivative1/1, Sum11/2
  Constant1/1 -> Sum2/2
  accel2force/1 -> Sum2/1
  Sum2/1 -> Saturation2/1
  Sum19/1 -> accel2force/1
  Mux5/1 -> Controllers 8/9
  Mux4/1 -> To Workspace5/1, Controllers 8/8
  Mux3/1 -> To Workspace4/1, Controllers 8/7
  Sum17/1 -> Sum15/1, Mux5/1  "desired_Az"
  actual_Az/1 -> Sum15/2, Band-limited Derivative10/1, Mux5/2
  actual_Vz/1 -> Band-limited Derivative9/1, Sum18/2, Mux4/2
  Mux1/1 -> To Workspace1/1, Controllers 8/2
  Mux/1 -> To Workspace/1, Controllers 8/1
  I_X8/1 -> Sum19/2
  Band-limited Derivative10/1 -> D_X8/1
  D_X8/1 -> Sum19/3
  P_X8/1 -> Sum19/1
  Integrator Limited10/1 -> I_X8/1, Display/1
  Sum15/1 -> P_X8/1, Integrator Limited10/1
  I_X7/1 -> Sum17/2
  Band-limited Derivative9/1 -> D_X7/1
  D_X7/1 -> Sum17/3
  P_X7/1 -> Sum17/1
  Integrator Limited9/1 -> I_X7/1, Display1/1
  Sum18/1 -> Integrator Limited9/1, P_X7/1
  I_X6/1 -> Sum20/2
  Band-limited Derivative8/1 -> D_X6/1
  actual_Pz/1 -> Sum16/2, Band-limited Derivative8/1, Mux3/2
  D_X6/1 -> Sum20/3
  P_X6/1 -> Sum20/1
  Integrator Limited8/1 -> I_X6/1
  Sum16/1 -> P_X6/1, Integrator Limited8/1
  desired_Py/1 -> Mux7/1, Sum13/1  "desired_Vy"
  I_X4/1 -> Sum12/2
  Band-limited Derivative6/1 -> D_X4/1
  D_X4/1 -> Sum12/3
  P_X4/1 -> Sum12/1
  Integrator Limited6/1 -> I_X4/1
  Sum13/1 -> P_X4/1, Integrator Limited6/1
  Band-limited Derivative1/1 -> D_X3/1
  P_X3/1 -> Sum4/1  "P"
  Integrator Limited1/1 -> I_X3/1
  Sum11/1 -> Integrator Limited1/1, P_X3/1
  Sum7/1 -> Controllers 8/3, Saturation/1  "desired_PITCH"
  desired_Px/1 -> Sum8/1, Mux1/1  "desired_Vx"
  I_X1/1 -> Sum7/2
  Band-limited Derivative4/1 -> D_X1/1
  actual_Vx/1 -> Band-limited Derivative4/1, Sum8/2, Mux1/2
  D_X1/1 -> Sum7/3
  P_X1/1 -> Sum7/1
  Integrator Limited4/1 -> I_X1/1
  Sum8/1 -> Integrator Limited4/1, P_X1/1
  Saturation2/1 -> altura_ctrl/1, Mux5/3  "altitude_control"
  I_X/1 -> Sum5/2
  Band-limited Derivative2/1 -> D_X/1
  actual_Px/1 -> Sum6/2, Band-limited Derivative2/1, Mux/2
  D_X/1 -> Sum5/3
  P_X/1 -> Sum5/1
  Integrator Limited3/1 -> I_X/1
  Sum6/1 -> P_X/1, Integrator Limited3/1
  Desired_Yaw/1 -> yaw_ctrl/1
  I_X3/1 -> Sum4/2  "I"
  D_X3/1 -> Sum4/3  "D"
  Clock/1 -> Sum/1
  Constant/1 -> Sum/2
  Sum/1 -> Switch/2
  Constant2/1 -> Switch/3
  Sum12/1 -> Switch/1
  Switch/1 -> P_pr1/1
  desired_Pz/1 -> Sum18/1, Mux4/1  "desired_Vz"

== system quad_sim_pyramid_formation/Quadrotor 8/Quadrirrotor Communication ==
  roll : Inport
  pitch : Inport  Port=2
  yaw : Inport  Port=3
  throttle : Inport  Port=4
  Blank Message : robotlib/Blank Message  SourceLibraryInfo=This block requires Robotics System Toolbox  messageType=geometry_msgs/Quaternion  SampleTime=inf
      settings: SourceProductBaseCode=RO
  Bus Assignment1 : BusAssignment  DialogController=Simulink.DDGSource_BusAssignment  AssignedSignals=X,Y,Z,W
  Bus Selector1 : BusSelector  OutputSignals=Data
  Data Type Conversion : DataTypeConversion  OutDataTypeStr=double
  Multiport Selector : dspindex/Multiport Selector  rowsOrCols=Rows  idxCellArray={ 1,2,3,4,5,6,7,8,9}  idxErrMode=Generate Error
  Publish2 : robotlib/Publish  SourceLibraryInfo=This block requires Robotics System Toolbox  topicSource=Specify your own  topic=/commands_attitude_8  messageType=geometry_msgs/Quaternion  messageQueueLength=105
      settings: SourceProductBaseCode=RO
  Subscribe : robotlib/Subscribe  SourceLibraryInfo=This block requires Robotics System Toolbox  topicSource=Specify your own  topic=/quadrotor_states_8  messageType=std_msgs/Float32MultiArray  sampleTime=-1  messageQueueLength=51
      settings: SourceProductBaseCode=RO
  Terminator : Terminator
  quad_pos_x : Outport
  quad_pos_y : Outport  Port=2
  quad_pos_z : Outport  Port=3
  quad_vel_x : Outport  Port=4
  quad_vel_y : Outport  Port=5
  quad_vel_z : Outport  Port=6
  quad_acc_x : Outport  Port=7
  quad_acc_y : Outport  Port=8
  quad_acc_z : Outport  Port=9
  wires:
  roll/1 -> Bus Assignment1/2
  pitch/1 -> Bus Assignment1/3
  yaw/1 -> Bus Assignment1/4
  throttle/1 -> Bus Assignment1/5
  Bus Selector1/1 -> Data Type Conversion/1  "<Data>"
  Data Type Conversion/1 -> Multiport Selector/1
  Multiport Selector/9 -> quad_acc_z/1
  Multiport Selector/8 -> quad_acc_y/1
  Multiport Selector/7 -> quad_acc_x/1
  Multiport Selector/6 -> quad_vel_z/1
  Multiport Selector/5 -> quad_vel_y/1
  Multiport Selector/4 -> quad_vel_x/1
  Multiport Selector/3 -> quad_pos_z/1
  Multiport Selector/2 -> quad_pos_y/1
  Multiport Selector/1 -> quad_pos_x/1
  Bus Assignment1/1 -> Publish2/1
  Subscribe/2 -> Bus Selector1/1
  Subscribe/1 -> Terminator/1
  Blank Message/1 -> Bus Assignment1/1

== system quad_sim_pyramid_formation/Quadrotor 8/Subsystem1 ==
  desired : Inport
  actual : Inport  Port=2
  roll_in : Inport  Port=3
  pitch_in : Inport  Port=4
  yaw_in : Inport  Port=5
  height_in : Inport  Port=6
  Clock : Clock
  Compare To Constant : simulink/Logic and Bit Operations/Compare To Constant  relop=<  const=0.5  OutDataTypeStr=boolean
  Compare To Constant1 : simulink/Logic and Bit Operations/Compare To Constant  relop=<=  const=0.025  OutDataTypeStr=boolean
  Compare To Zero : simulink/Logic and Bit Operations/Compare To Zero  relop=<=  OutDataTypeStr=boolean
  Constant : Constant  Value=0
  Constant1 : Constant
  Data Store Memory : DataStoreMemory  DataStoreName=waypoints_reached8  ShowAdditionalParam=off  OutDataTypeStr=boolean
  Data Store Read{,1..4} (5 alike) : DataStoreRead  DataStoreName=waypoints_reached8
  Data Store Write : DataStoreWrite  DataStoreName=waypoints_reached8
  Demux : Demux  Outputs=3
  Fcn : Fcn  Expr=sqrt(u(1)^2+u(2)^2+u(3)^2)
  Logical Operator : Logic  AllPortsSameDT=off  OutDataTypeStr=boolean
  Mux8 : Mux  Inputs=3
  Sum1 : Sum  Inputs=+-
  Switch{,1..4} (5 alike) : Switch  Criteria=u2 > Threshold  Threshold=0.5
  Switch5 : Switch  Criteria=u2 > Threshold  Threshold=time_to_enable
  "angle " : Constant  Value=0
  angle 1 : Constant  Value=0
  angle 2 : Constant  Value=0
  angle 3 : Constant  Value=-1
  roll_out : Outport
  pitch_out : Outport  Port=2
  yaw_out : Outport  Port=3
  height_out : Outport  Port=4
  wires:
  roll_in/1 -> Switch1/3
  pitch_in/1 -> Switch2/3
  angle 2/1 -> Switch3/1
  yaw_in/1 -> Switch3/3
  "angle "/1 -> Switch1/1
  angle 1/1 -> Switch2/1
  height_in/1 -> Switch4/3
  Switch2/1 -> pitch_out/1
  Switch1/1 -> roll_out/1
  Demux/2 -> Mux8/2
  Demux/3 -> Switch5/1, Mux8/3
  Logical Operator/1 -> Switch/3
  Compare To Constant/1 -> Logical Operator/1
  Compare To Constant1/1 -> Logical Operator/2
  Sum1/1 -> Fcn/1
  Fcn/1 -> Compare To Constant1/1
  Mux8/1 -> Sum1/1
  Compare To Zero/1 -> Switch/1
  Data Store Read2/1 -> Switch2/2
  Data Store Read4/1 -> Switch4/2
  Data Store Read1/1 -> Switch1/2
  Switch/1 -> Data Store Write/1
  Data Store Read3/1 -> Switch3/2
  angle 3/1 -> Switch4/1
  Switch3/1 -> yaw_out/1
  Switch4/1 -> height_out/1
  Data Store Read/1 -> Switch/2
  Constant/1 -> Compare To Zero/1
  Demux/1 -> Mux8/1
  desired/1 -> Demux/1
  actual/1 -> Sum1/2
  Clock/1 -> Switch5/2
  Constant1/1 -> Switch5/3
  Switch5/1 -> Compare To Constant/1
